simulink model "Delta_robot2019B"  (R2019b)
settings: Solver=VariableStepAuto  StartTime=0.0  StopTime=10.0  RelTol=1e-3
model workspace: external: MATLAB File C:\Users\rpk16\Documents\Mechatronics System Lab\Delta robot Simulink\Delta_robot_assembly_DataFile.m (data not in the file)
undefined symbols (not defined in the file or in its folder): _Default_sldprt, delta_arm_spherical_joint, delta_link1, smiData, X, Y, Z
libraries: sm_lib x144, nesl_utility x7, simulink x4
(part 4 of 4)

== matlab function Delta_robot2019B/Motion Control ==
  data: M3 output; M2 output; Signal input; M1 output; option input
function [M3,M2,M1] = fcn(Signal,option)
Speed = pi/40;
switch(option)    
    case 1
        M1 = Signal*Speed;
        M2 = Signal*Speed;
        M3 = Signal*Speed;
    case 2
        M1 = Signal*-Speed;
        M2 = Signal*-Speed;
        M3 = Signal*-Speed;
    case 3
        M1 = Signal*Speed;
        M2 = Signal*Speed;
        M3 = Signal*-Speed;
    case 4
        M1 = Signal*-Speed;
        M2 = Signal*-Speed;
        M3 = Signal*Speed;
    case 5
        M1 = Signal*-Speed;
        M2 = Signal*Speed;
        M3 = Signal*-Speed;
    case 6
        M1 = Signal*Speed;
        M2 = Signal*-Speed;
        M3 = Signal*-Speed;
    otherwise
        M1 = 0;
        M2 = 0;
        M3 = 0;        
end
end
